simulink model "target_udp_comm1"  (Simulink 7.3)
settings: Solver=FixedStepDiscrete  SolverMode=SingleTasking  StartTime=0.0  StopTime=10.0  RelTol=1e-3
PreLoadFcn:
  | waijung.modelPreload; % Required for working with Waijung Blockset. Do not remove.
undefined symbols (not defined in the file): A0, A1, A2, A3, A7, B0, B1, B10, B11, B12, B13, C1, C2, C3, C4, C5, HSEOSC, Link, LQFP176, ST, STM32F417IG
libraries: stm32f4_io_lib x2, waijung_webserver x2, waijung_socket_lib x2, stm32f4_device_config_lib x1
CloseFcn:
  | waijung.modelClose; % Required for working with Waijung Blockset. Do not remove.
settings Model: Creator=Krisada  LastModifiedBy=Krisada
settings OptimizationCC: OptimizeModelRefInitCode=on  LifeSpan=1
settings HardwareCC: ProdEndianess=LittleEndian  ProdHWDeviceType=ARM Compatible->Cortex - M4  TargetEndianess=LittleEndian  TargetHWDeviceType=ARM Compatible->Cortex - M4
settings RTWCC: SystemTargetFile=stm32f4.tlc  GenerateMakefile=off  TemplateMakefile=ert_default_tmf  Description=STM32F4 Target  ProcessScript=stm32f4_make_rtw_hook
settings CodeAppCC: IgnoreCustomStorageClasses=off
settings STFCustomTargetCC: ModelReferenceCompliant=off  CombineOutputUpdateFcns=on  ERTCustomFileBanners=on  SupportContinuousTime=off  SupportNonInlinedSFcns=off  SystemTargetFile=stm32f4.tlc
settings ERTTargetCC: MultiwordLength=2048  ModelReferenceCompliant=off  ParMdlRefBuildCompliant=off  CompOptLevelCompliant=off  ERTFirstTimeCompliant=off  ModelStepFunctionPrototypeControlCompliant=off  CPPClassGenCompliant=off  ExtModeMexFile=noextcomm  InlinedParameterPlacement=NonHierarchical  ERTSrcFileBannerTemplate=stm32f4_code_template.cgt  ERTHdrFileBannerTemplate=stm32f4_code_template.cgt  ERTDataSrcFileTemplate=stm32f4_code_template.cgt  ERTDataHdrFileTemplate=stm32f4_code_template.cgt  ERTCustomFileTemplate=stm32f4_file_process.tlc

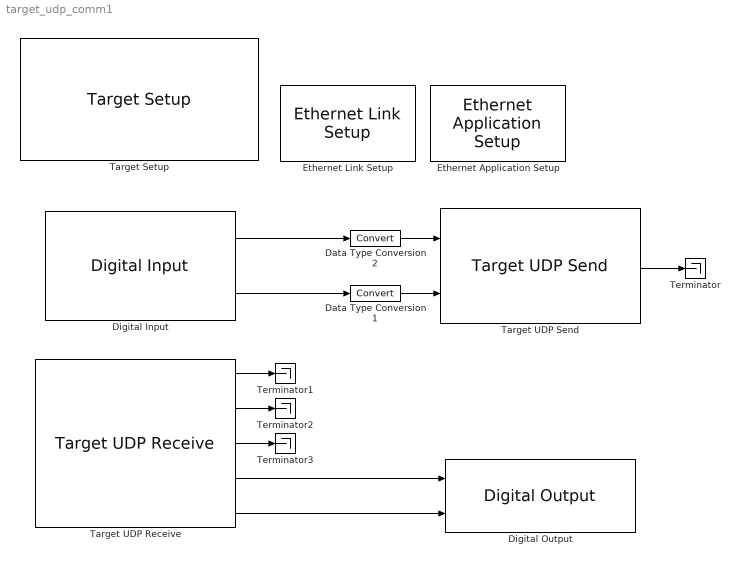
== system target_udp_comm1 ==
  Data Type Conversion1 : DataTypeConversion  OutDataType=fixdt(1, 16)  OutScaling=2^0
  Data Type Conversion2 : DataTypeConversion  OutDataType=fixdt(1, 16)  OutScaling=2^0
  Digital Input : stm32f4_io_lib/Digital Input  port=B  speed=100  porttype=None  porttypestr=NOPULL  use_pin0=off  use_pin1=off  use_pin2=on  use_pin3=off  use_pin4=off  use_pin5=off  use_pin6=off  use_pin7=off  use_pin8=off  use_pin9=off  use_pin10=off  use_pin11=off  use_pin12=off  use_pin13=off  use_pin14=off  use_pin15=on  pinstr=GPIO_Pin_2 | GPIO_Pin_15  usedpinarray="[0  0  1  0  0  0  0  0  0  0  0  0  0  0  0  1]"  bitbandingstr=|  sampletime=0.001  sampletimestr=0.001  blockid=DigitalInput  enablecustomportlabel=off  glabalinit=off  cinputportlabel=In1, In2  coutputportlabel=Out1, Out2
      | #define DigitalInput_B2 Peripheral_BB(GPIOB->IDR, 2)  /* Output pin */
      | #define DigitalInput_B15 Peripheral_BB(GPIOB->IDR, 15)  /* Output pin */
  Digital Output : stm32f4_io_lib/Digital Output  use_bitband=on  port=D  speed=100  porttype=Push Pull  porttypestr=PP  use_pin0=off  use_pin1=off  use_pin2=off  use_pin3=off  use_pin4=off  use_pin5=off  use_pin6=off  use_pin7=off  use_pin8=off  use_pin9=off  use_pin10=off  use_pin11=off  use_pin12=on  use_pin13=on  use_pin14=off  use_pin15=off  pinstr=GPIO_Pin_12 | GPIO_Pin_13  usedpinarray="[0  0  0  0  0  0  0  0  0  0  0  0  1  1  0  0]"  bitbandingstr=|  sampletime=-1  sampletimestr=0.0001  blockid=DigitalOutput  enablecustomportlabel=off  globalinit=off  cinputportlabel=In1, In2  coutputportlabel=0
      | #define DigitalOutput_D12 Peripheral_BB(GPIOD->ODR, 12)  /* Output pin */
      | #define DigitalOutput_D13 Peripheral_BB(GPIOD->ODR, 13)  /* Output pin */
  Ethernet Application Setup : waijung_webserver/Ethernet Application Setup  conf=Setup  ipaddress=192.168.1.31  netmask=255.255.255.0  gateway=192.168.1.1  macaddress=02-00-00-00-00-00  dhcp=off  timerscaler=10  portpinstr=0  sampletime=0.0001  blockid=EthernetApplicationSetup  inputporttype=[]  inputportwidth=[]  inputportlabel={}  outputporttype=[]  outputportwidth=[]  outputportlabel={}  compat=0  optionstring="[\"Dummy\",\"192\",\"168\",\"1\",\"31\",\"255\",\"255\",\"255\",\"0\",\"192\",\"168\",\"1\",\"1\",\"02\",\"00\",\"00\",\"00\",\"00\",\"00\",\"off\",\"10\"]"
  Ethernet Link Setup : waijung_webserver/Ethernet Link Setup  conf=Setup  interfacepin=Profile #1  wj_interfacetype=MII  pin_mdio=A2  pin_mdc=C1  pin_pps=Not used  pin_crs=A0  pin_col=A3  pin_dv=A7  pin_rxclk=A1  pin_rxer=B10  pin_rxd0=C4  pin_rxd1=C5  pin_rxd2=B0  pin_rxd3=B1  pin_txclk=C3  pin_txen=B11  pin_txd0=B12  pin_txd1=B13  pin_txd2=C2  pin_txd3=E2  portpinstr=A0,A1,A2,A3,A7,B0,B1,E2,B10,B11,B12,B13,C1,C2,C3,C4,C5  sampletime=inf  blockid=EthernetLinkSetup  inputporttype=[]  inputportwidth=[]  inputportlabel={}  outputporttype=[]  outputportwidth=[]  outputportlabel={}  compat=0  optionstring="[\"xxx\",\"on\",\"on\",\"on\",\"off\",\"on\",\"off\",\"off\",\"off\",\"off\",\"on\",\"on\",\"on\",\"on\",\"on\",\"on\",\"on\",\"off\",\"on\",\"on\",\"on\",\"on\",\"on\",\"on\",\"on\",\"on\",\"on\",\"on\",\"A\",\"0\",\"A\",\"1\",\"A\",\"2\",\"A\",\"3\",\"A\",\"7\",\"B\",\"0\",\"B\",\"1\",\"N\",\"ot used\",\"E\",\"2\",\"B\",\"10\",\"B\",\"11\",\"B\",\"12\",\"B\",\"13\",\"C\",\"1\",\"C\",\"2\",\"C\",\"3\",\"C\",\"4\",\"C\",\"5\",\"MII\"]"
  Target Setup : stm32f4_device_config_lib/Target Setup  Priority=100  compiler=GNU ARM  previous_compiler=GNU ARM  mcu=STM32F417IG (LQFP176)  mcustr=STM32F417IG  clockconfig=HSEOSC-8MHz  system_stm32f4xx_c_path=F:\trunk\targets\stm32f4_target\stm32f4\utils\system_stm32f4xx_default\STM32F40_41xxx\hseosc8mhz  showmemoryconfiguration=off  stacksize=0x2000  heapsize=0x2000  enableautocompiledownload=on  fullchiperase=off  programmerinterface=ST-Link  editctrlstr=on  compilercontrolstr=$(patsubst %, -I%, .) -mcpu=cortex-m4 -mthumb -mthumb-interwork -mfloat-abi=hard -mfpu=fpv4-sp-d16 -ffast-math -Wall -Wextra -Ofast  assemblercontrolstr=$(patsubst %, -I%, .) -mcpu=cortex-m4 -mthumb -mthumb-interwork -mfloat-abi=hard -mfpu=fpv4-sp-d16 -ffast-math -Wall -Wextra -Ofast -Wa,-amhls=$(<:.s=.lst) -D__STACK_SIZE=$(STACK_SIZE) -D__HEAP_SIZE=$(HEAP_SIZE)  linkercontrolstr=-T$(LD_SCRIPT) -g -Wl,-Map=$(MAP),--cref,--no-warn-mismatch -mcpu=cortex-m4 -mthumb -mthumb-interwork -mfloat-abi=hard -mfpu=fpv4-sp-d16 -specs=nosys.specs  runafterdownload=on  execprofile=None  profileruart=3  profilerbaud=500000  profilertxpin=D8  profilerinitstr=0.0001,168000000,16800,500000,0  manualsetsampletime=off  sampletime=0.0001  blockid=TargetSetup  systickreloadvalue=16800  hseval=8000000  lastprofileruart=3  hclk=168000000  flashorigin=0x8000000  flashlength=1024k  ramorigin=0x20000000  ramlength=128k  useextram=off
  Target UDP Receive : waijung_socket_lib/Target UDP Receive  conf=TargetReceive  protocol=UDP  port=7  address=192.168.1.21  echo=off  transfer=Non-blocking  timeout=5  datasource=Ports  datatype=uint8  datacount=2  porttype_double=0  porttype_single=0  porttype_int8=0  porttype_uint8=2  porttype_int16=0  porttype_uint16=0  porttype_int32=0  porttype_uint32=0  portpinstr=0  sampletime=inf  blockid=TargetUDPReceive  inputporttype=[]  inputportwidth=[]  inputportlabel={}  outputporttype=[7,5,3,3,3]  outputportwidth=[1,1,4,]  outputportlabel={'Status','Remote Port','Remote IP(1:4)','uint8 D0','uint8 D1'}  compat=0  optionstring="[\"UDP\",\"7\",\"192\",\"168\",\"1\",\"21\",\"Non-blocking\",\"PortData\",\"uint8_t\",\"2\",\"Receive\",\"off\",\"\",\"\",\"\",\"\",\"\",\"\",\"\"]"  options=[7,2,1,5000,0]
  Target UDP Send : waijung_socket_lib/Target UDP Send  conf=TargetSend  protocol=UDP  variableipport=off  port=7  address=192.168.1.41  echo=off  transfer=Non-blocking  timeout=5  datasource=Ports  streamsource=ExtRAM  streamsize=512  datatype=uint8  datacount=2  porttype_double=0  porttype_single=0  porttype_int8=0  porttype_uint8=2  porttype_int16=0  porttype_uint16=0  porttype_int32=0  porttype_uint32=0  portpinstr=0  sampletime=-1  blockid=TargetUDPSend  inputporttype=[3,3]  inputportwidth=[1]  inputportlabel={'D0 uint8','D1 uint8'}  outputporttype=[7]  outputportwidth=[]  outputportlabel={'Status'}  compat=0  optionstring="[\"UDP\",\"7\",\"192\",\"168\",\"1\",\"41\",\"Non-blocking\",\"PortData\",\"uint8_t\",\"2\",\"Send\",\"off\",\"off\",\"\",\"\",\"\",\"\",\"\",\"512\"]"  options=[7,2,0,5000,0]
  Terminator{,1..3} (4 alike) : Terminator
  wires:
  Target UDP Send/1 -> Terminator/1
  Target UDP Receive/1 -> Terminator1/1
  Target UDP Receive/2 -> Terminator2/1
  Target UDP Receive/3 -> Terminator3/1
  Digital Input/2 -> Data Type Conversion1/1
  Target UDP Receive/4 -> Digital Output/1
  Target UDP Receive/5 -> Digital Output/2
  Data Type Conversion2/1 -> Target UDP Send/1
  Data Type Conversion1/1 -> Target UDP Send/2
  Digital Input/1 -> Data Type Conversion2/1
